simulink model "adc_lib2"  (R2018b)
settings: Solver=ode45  StartTime=0.0  StopTime=10e-05  RelTol=1e-3  EnableMultiTasking=on
libraries: mylib2 x1, dsparch4 x1
settings Model: Creator=bbhattac  LastModifiedBy=khung
settings DataIOCC: LimitDataPoints=on  SaveFormat=Array
settings OptimizationCC: ExpressionDepthLimit=2147483647  LifeSpan=inf
settings DebuggingCC: UnderspecifiedInitializationDetection=Classic  MergeDetectMultiDrivingBlocksExec=none  SolverPrmCheckMsg=warning  ParameterPrecisionLossMsg=none  FcnCallInpInsideContextMsg=warning  StateNameClashWarn=warning  SFUnexpectedBacktrackingDiag=warning  SFNoUnconditionalDefaultTransitionDiag=warning  SFExecutionAtInitializationDiag=none
settings HardwareCC: ProdBitPerPointer=32  ProdBitPerSizeT=32  ProdBitPerPtrDiffT=32  ProdLargestAtomicFloat=None  ProdIntDivRoundTo=Undefined  ProdEndianess=Unspecified  ProdWordSize=32  ProdHWDeviceType=32-bit Generic
settings ModelReferenceCC: PropagateSignalLabelsOutOfModel=off
settings SFSimCC: SimUseLocalCustomCode=off
settings RTWCC: RTWUseLocalCustomCode=off
settings CodeAppCC: StateflowObjectComments=on
settings GRTTargetCC: TargetLangStandard=C89/C90 (ANSI)  GeneratePreprocessorConditionals=Disable all  CombineOutputUpdateFcns=off  GRTInterface=on
settings ConfigComp: CovMetricSettings=dw  CovHtmlReporting=on  CovSaveCumulativeToWorkspaceVar=on  CovSaveSingleToWorkspaceVar=on  CovExternalEMLEnable=off

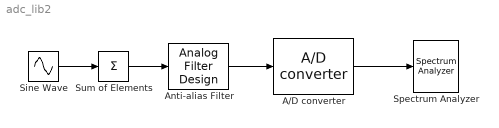
== system adc_lib2 ==
  A/D converter : mylib2/A//D converter  minDelay=1.0e-09  maxDelay=15.0e-09  nonlingain=0.2  nbits=8
  Anti-alias Filter : dsparch4/Analog Filter Design  method=Butterworth  filttype=Lowpass  N=8  Wlo=2*pi*50e+06  Whi=80  Rp=2  Rs=40
  Sine Wave : Sin  Amplitude=.5  Frequency=2*pi*[20 22]*1e6  SampleTime=0
  Spectrum Analyzer : SpectrumAnalyzer
  Sum of Elements : Sum  Inputs=+
  wires:
  Sine Wave/1 -> Sum of Elements/1
  Sum of Elements/1 -> Anti-alias Filter/1
  Anti-alias Filter/1 -> A/D converter/1
  A/D converter/1 -> Spectrum Analyzer/1
